simulink model "tram_sim"  (R2019b)
settings: Solver=VariableStepAuto  StartTime=0.0  StopTime=700  RelTol=1e-3
values from neighbouring files (symbols this model uses):
  B = 1/3*Te_n*1/w_b    (= 1.3022339824)    [tram.m]
  e_n = Ks*ie_max*w_b    (= 540)    [tram.m]
  g = 9.81    [tram.m]
  ie_max = 1    [tram.m]
  J = m_t*r_whl^2    (= 73.2506615098)    [tram.m]
  kb_a = 1/tau_a    (= 100)    [tram.m]
  kb_e = 1/tau_e    (= 1)    [tram.m]
  kb_spd = 1/tau_s    (= 5)    [tram.m]
  Kie = Ci_e.Ki    [tram.m]
  Kim = Cm.Ki    [tram.m]
  Kpe = Ci_e.Kp    [tram.m]
  Kpm = Cm.Kp    [tram.m]
  Ks = v_line*eta/(ie_max*w_b)    (= 1.71974522293)    [tram.m]
  La = tau_a*Ra    (= 0.00104347826087)    [tram.m]
  Le = tau_e*Re    (= 120)    [tram.m]
  m_t = m_train + m_load    (= 26000)    [tram.m]
  r_whl = s_b/w_b*10/36    (= 0.0530785562633)    [tram.m]
  Ra = (v_line-e_n)/ia_n    (= 0.104347826087)    [tram.m]
  Re = ve_max/ie_max    (= 120)    [tram.m]
  s_b = 60    [tram.m]
  Te_n = 4/3*F_tr*r_whl    (= 1226.70441142)    [tram.m]
  v_line = 600    [tram.m]
  ve_max = 120    [tram.m]
  w_b = 314    [tram.m]
undefined symbols (not defined in the file or in its folder): sigbuilder_block
settings Model: Creator=hassancurrimbhoy  LastModifiedBy=hassancurrimbhoy
settings SolverCC: ZeroCrossAlgorithm=Adaptive
settings DebuggingCC: IgnoredZcDiagnostic=none

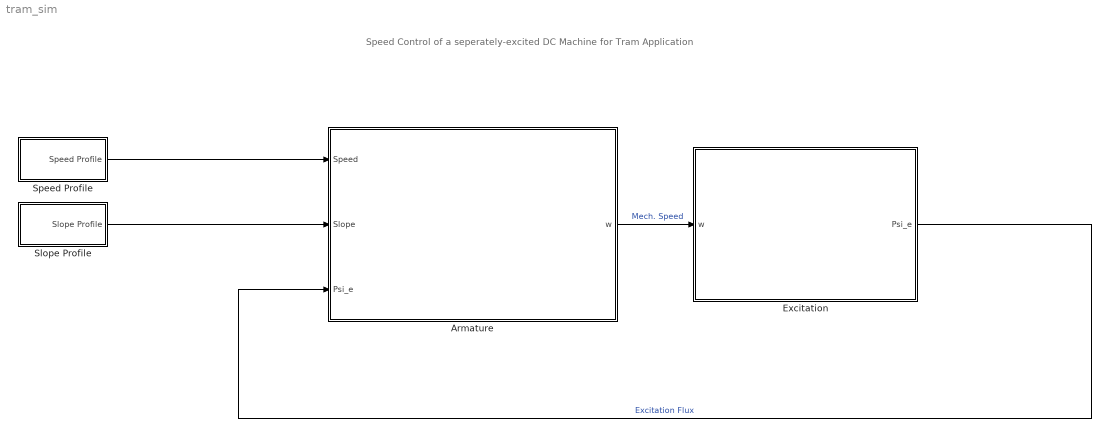
== system tram_sim ==
  note: Speed Control of a seperately-excited DC Machine for Tram Application
  Armature : Subsystem
  Excitation : Subsystem
  Slope Profile : Subsystem  Tag=STV Subsys  LoadFcn=sigbuilder_block('load');  StartFcn=sigbuilder_block('start');  StopFcn=sigbuilder_block('stop');  ClipboardFcn=sigbuilder_block('clipboard');  mask(Sigbuilder block){tuvar=[0:10]}
      mask help: Simulink:masks:SigbuilderBlock_MD
      mask init:
      | if ~strcmp(get_param(bdroot(gcbh),'SimulationStatus'),'stopped') tuvar = sigbuilder_block('maskInit'); end
      settings: CopyFcn=sigbuilder_block('copy');  DeleteFcn=sigbuilder_block('delete');  ModelCloseFcn=sigbuilder_block('modelClose');  PreSaveFcn=sigbuilder_block('preSave');  PauseFcn=sigbuilder_block('pause');  ContinueFcn=sigbuilder_block('continue');  NameChangeFcn=sigbuilder_block('namechange');  OpenFcn=sigbuilder_block('open',[437.6 199.2 550.4 400 ]);  CloseFcn=sigbuilder_block('close');
      mask Display: plot(0, 0, 100, 100,[2, 2, 32, 32, 2], [68, 8, 8, 68, 68],[32, 2], [38, 38], [32, 19, 2],[53, 60, 44], [32, 17, 17, 2],[16, 16, 31, 31]);txt = getActiveGroup(gcbh);text(2, 100, txt,'verticalAlignment', 'top');
  Speed Profile : Subsystem  Tag=STV Subsys  LoadFcn=sigbuilder_block('load');  StartFcn=sigbuilder_block('start');  StopFcn=sigbuilder_block('stop');  ClipboardFcn=sigbuilder_block('clipboard');  mask(Sigbuilder block){tuvar=[0:10]}
      mask help: Simulink:masks:SigbuilderBlock_MD
      mask init:
      | if ~strcmp(get_param(bdroot(gcbh),'SimulationStatus'),'stopped') tuvar = sigbuilder_block('maskInit'); end
      settings: CopyFcn=sigbuilder_block('copy');  DeleteFcn=sigbuilder_block('delete');  ModelCloseFcn=sigbuilder_block('modelClose');  PreSaveFcn=sigbuilder_block('preSave');  PauseFcn=sigbuilder_block('pause');  ContinueFcn=sigbuilder_block('continue');  NameChangeFcn=sigbuilder_block('namechange');  OpenFcn=sigbuilder_block('open',[437.6 199.2 550.4 400 ]);  CloseFcn=sigbuilder_block('close');
      mask Display: plot(0, 0, 100, 100,[2, 2, 32, 32, 2], [68, 8, 8, 68, 68],[32, 2], [38, 38], [32, 19, 2],[53, 60, 44], [32, 17, 17, 2],[16, 16, 31, 31]);txt = getActiveGroup(gcbh);text(2, 100, txt,'verticalAlignment', 'top');
  wires:
  Excitation/1(Psi_e) -> Armature/3(Psi_e)  "Excitation Flux"
  Armature/1(w) -> Excitation/1(w)  "Mech. Speed"
  Slope Profile/1(Slope Profile) -> Armature/2(Slope)
  Speed Profile/1(Speed Profile) -> Armature/1(Speed)

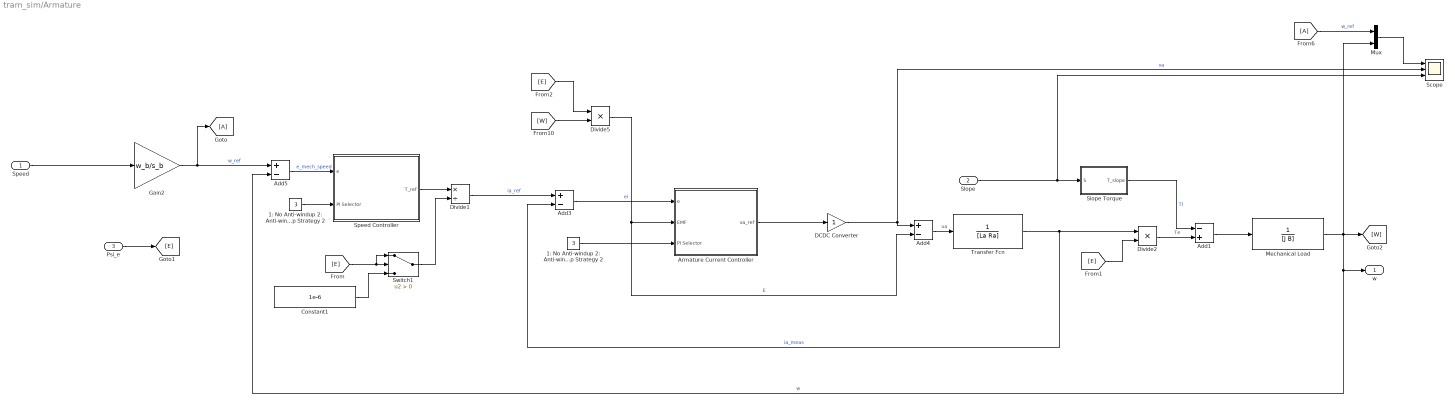
== system tram_sim/Armature ==
  Speed : Inport
  Slope : Inport  Port=2
  Psi_e : Inport  Port=3
  1: No Anti-windup 2: Anti-windup Stragtegy 1 3: Anti-windup Strategy 2 : Constant  Value=3
  1: No Anti-windup 2: Anti-windup Strategy 1 3: Anti-windup Strategy 2 : Constant  Value=3
  Add1 : Sum  Inputs=-+
  Add3 : Sum  Inputs=+-
  Add4 : Sum  Inputs=+-
  Add5 : Sum  Inputs=+-
  Armature Current Controller : Subsystem
  Constant1 : Constant  Value=1e-6
  DCDC Converter : Gain
  Divide1 : Product  Inputs=*/
  Divide2 : Product  Inputs=**
  Divide5 : Product  Inputs=**
  Gain2 : Gain  Gain=w_b/s_b
  Mechanical Load : TransferFcn  Denominator=[J B]
  Mux : Mux  Inputs=2
  Scope : Scope  NumInputPorts=3
  Slope Torque : Subsystem
  Speed Controller : Subsystem
  Switch1 : Switch  Criteria=u2 > Threshold
  Transfer Fcn : TransferFcn  Denominator=[La Ra]
  w : Outport
  wires:
  1: No Anti-windup 2: Anti-windup Stragtegy 1 3: Anti-windup Strategy 2/1 -> Speed Controller/2(PI Selector)
  Armature Current Controller/1("va_ref ") -> DCDC Converter/1
  Constant1/1 -> Switch1/3
  Add1/1 -> Mechanical Load/1
  Gain2/1 -> Add5/1, [A]  "w_ref"
  Mechanical Load/1 -> Mux/2, [W], w/1, Add5/2  "w"
  [A] -> Mux/1  "w_ref"
  [W] -> Divide5/2
  Mux/1 -> Scope/1
  Slope Torque/1(T_slope) -> Add1/1  "Tl"
  Add5/1 -> Speed Controller/1(e)  "e_mech_speed"
  Speed Controller/1("T_ref ") -> Divide1/1
  DCDC Converter/1 -> Scope/2, Add4/1  "va"
  Divide2/1 -> Add1/2  "Te"
  Add3/1 -> Armature Current Controller/1(e)  "ei"
  Add4/1 -> Transfer Fcn/1  "ua"
  [E] -> Divide2/2
  1: No Anti-windup 2: Anti-windup Strategy 1 3: Anti-windup Strategy 2/1 -> Armature Current Controller/3("PI Selector ")
  Divide1/1 -> Add3/1  "ia_ref"
  Divide5/1 -> Add4/2, Armature Current Controller/2(EMF)  "E"
  [E] -> Switch1/1, Switch1/2
  Transfer Fcn/1 -> Divide2/1, Add3/2  "ia_meas"
  Psi_e/1 -> [E]
  [E] -> Divide5/1
  Speed/1 -> Gain2/1
  Slope/1 -> Scope/3, Slope Torque/1(S)
  Switch1/1 -> Divide1/2

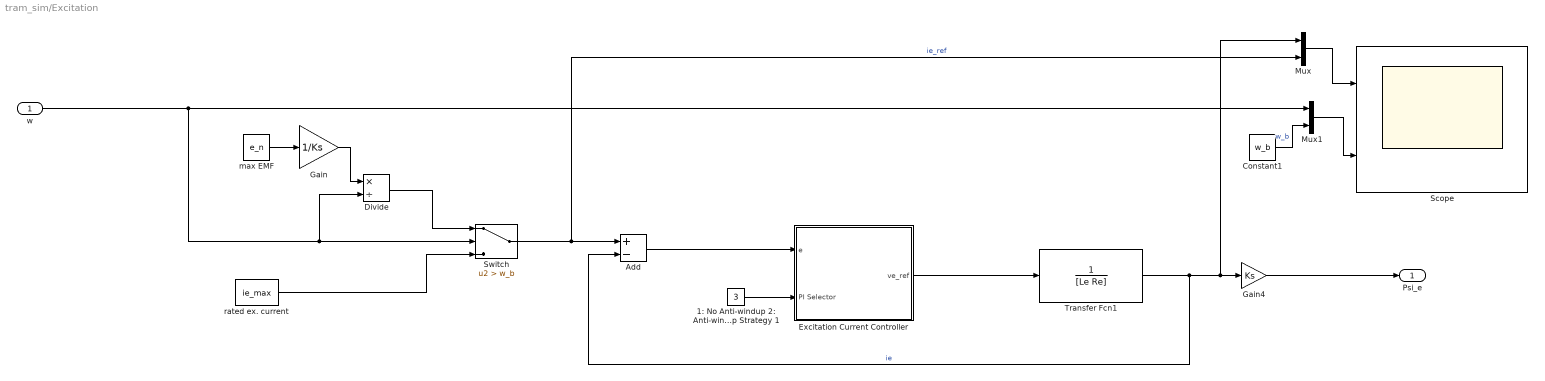
== system tram_sim/Excitation ==
  w : Inport
  1: No Anti-windup 2: Anti-windup Strategy 1 3: Anti-windup Strategy 1 : Constant  Value=3
  Add : Sum  Inputs=+-
  Constant1 : Constant  Value=w_b
  Divide : Product  Inputs=*/
  Excitation Current Controller : Subsystem
  Gain : Gain  Gain=1/Ks
  Gain4 : Gain  Gain=Ks
  Mux : Mux  Inputs=2
  Mux1 : Mux  Inputs=2
  Scope : Scope  NumInputPorts=2
  Switch : Switch  Criteria=u2 > Threshold  Threshold=w_b
  Transfer Fcn1 : TransferFcn  Denominator=[Le Re]
  max EMF : Constant  Value=e_n
  rated ex. current : Constant  Value=ie_max
  Psi_e : Outport
  wires:
  Excitation Current Controller/1("ve_ref ") -> Transfer Fcn1/1
  Add/1 -> Excitation Current Controller/1(e)
  Gain/1 -> Divide/1
  Transfer Fcn1/1 -> Mux/1, Gain4/1, Add/2  "ie"
  rated ex. current/1 -> Switch/3
  1: No Anti-windup 2: Anti-windup Strategy 1 3: Anti-windup Strategy 1/1 -> Excitation Current Controller/2("PI Selector ")
  Switch/1 -> Mux/2, Add/1  "ie_ref"
  Divide/1 -> Switch/1
  max EMF/1 -> Gain/1
  w/1 -> Switch/2, Divide/2, Mux1/1
  Mux/1 -> Scope/1
  Constant1/1 -> Mux1/2  "w_b"
  Mux1/1 -> Scope/2
  Gain4/1 -> Psi_e/1

== system tram_sim/Slope Profile ==
  Demux : Demux  Tag=STV Demux  Outputs=1
  FromWs : FromWorkspace  Tag=STV FromWs  VariableName=tuvar  SampleTime=0
      SigBuilderData=|
      | common.afterFinalStr = 'Extrapolate'
      | common.sampleTime = 0
      | dataSet.timeRange = [0 700]
      | dataSet.name = 'Group 1'
      | sbobj.Groups.Name = 'Group 1'
      | sbobj.Groups.Signals.Name = 'Slope Profile'
      | sbobj.Groups.Signals.XData = [0 1 2 3 4 5 6 7 8 9 10 11 ... (662 elements, 1x662)]
      | sbobj.Groups.Signals.YData = [0 0 0 0 0 0 0 0 0 0 0 0 0 0 0 0 0 0 0 0 0 0 0 0 0 0 0 0 0 0 0 0 0 0 0 0 0 0 0 0 0 0 0 0 0 0 0 0 0 0 0 0 0 0 0 0 0 0 0 0 0 0 0 0 0 0 0 0 0 0 0 0 0 0 0 0 0 0 0 0 0 0 0 0 0 0 0 0 0 0 0 0 0 0 0 0 0 0 0 0 0 0 0 0 0 0 0 0 0 0 0 0 0 0 0 0 0 0 0 0 0 0 0 0 0 0 0 0 0 0 0 0 0 0 0 0 0 0 0 0 0 0 0 0 0 0 0 0 0 0 0 0 0 0 0 0 0 0 0 0 0 0 0 0 0 0 0 0 0 0 0 0 0 0 0 0 0 0 0 0 0 0 0 0 0 0 0 0 0 0 0 0 0 0 0 0 0 0 0 0 0 0 0 0 0 0 0 0 0 0 0 0 0 0 0 0 0 0 0 0 0 0 0 5 5 5 5 5 5 5 5 5 5 5 5 5 5 5 5 5 5 5 5 5 5 5 5 5 5 5 5 5 5 5 5 5 5 5 5 5 5 5 5 5 5 5 5 5 5 5 5 5 5 5 5 5 5 5 5 5 5 5 5 0 0 0 0 0 0 0 0 0 0 0 0 0 0 0 0 0 0 0 0 0 0 0 0 0 0 0 0 0 0 0 0 0 0 0 0 0 0 0 0 0 0 0 0 0 0 0 0 0 0 0 0 0 0 0 0 0 0 0 0 0 0 0 0 0 0 0 0 0 0 0 0 0 0 0 0 0 0 0 0 0 0 0 0 0 0 0 0 0 0 0 0 0 0 0 0 0 0 0 0 0 0 0 0 0 0 0 0 0 0 0 0 0 0 0 0 0 0 0 0 0 0 0 0 0 0 0 0 0 0 0 0 0 0 0 0 0 0 0 0 0 0 0 0 0 0 0 0 0 0 0 0 0 0 0 0 0 0 0 0 0 0 0 0 0 0 0 0 0 0 0 0 0 0 0 0 0 0 0 0 0 0 0 0 0 0 0 0 0 0 0 0 0 0 0 0 0 0 0 0 0 0 0 0 0 0 0 0 0 0 0 0 0 0 0 0 -5 -5 -5 -5 -5 -5 -5 -5 -5 -5 -5 -5 -5 -5 -5 -5 -5 -5 -5 -5 -5 -5 -5 -5 -5 -5 -5 -5 -5 -5 -5 -5 -5 -5 -5 -5 -5 -5 -5 -5 -5 -5 -5 -5 -5 -5 -5 -5 -5 -5 -5 -5 -5 -5 -5 -5 -5 -5 -5 -5 0 0 0 0 0 0 0 0 0 0 0 0 0 0 0 0 0 0 0 0 0 0 0 0 0 0 0 0 0 0 0 0 0 0 0 0 0 0 0 0 0 0 0 0 0 0 0 0 0 0 0 0 0 0 0 0 0 0 0 0 0 0 0 0 0 0 0 0 0 0 0 0 0 0 0 0 0 0 0 0 0 0 0 0 0 0 0 0 0 0 0 0 0 0 0 0 0 0 0 0 0 0 0]
      | sbobj.Groups.TimeRange = [0 700]
  Slope Profile : Outport  Tag=STV Outport
  wires:
  FromWs/1 -> Demux/1
  Demux/1 -> Slope Profile/1

== system tram_sim/Speed Profile ==
  Demux : Demux  Tag=STV Demux  Outputs=1
  FromWs : FromWorkspace  Tag=STV FromWs  VariableName=tuvar  SampleTime=0
      SigBuilderData=|
      | common.afterFinalStr = 'Extrapolate'
      | common.sampleTime = 0
      | dataSet.timeRange = [0 700]
      | dataSet.name = 'Group 1'
      | sbobj.Groups.Name = 'Group 1'
      | sbobj.Groups.Signals.Name = 'Speed Profile'
      | sbobj.Groups.Signals.XData = [0 1 2 3 4 5 6 7 8 9 10 11 ... (662 elements, 1x662)]
      | sbobj.Groups.Signals.YData = [35 35 35 35 35 35 35 35 35 35 35 35 35 35 35 35 35 35 35 35 35 35 35 35 35 35 35 35 35 35 35 35 35 35 35 35 35 35 35 35 35 35 35 35 35 35 35 35 35 35 35 35 35 35 35 35 35 35 35 35 35 35 35 35 35 35 35 35 35 35 35 35 35 35 35 35 35 35 35 35 35 35 35 35 35 35 35 35 35 35 35 35 35 35 35 35 35 35 35 35 35 35 35 60 60 60 60 60 60 60 60 60 60 60 60 60 60 60 60 60 60 60 60 60 60 60 60 60 60 60 60 60 60 60 60 60 60 60 60 60 60 60 60 60 60 60 60 60 60 60 60 60 60 60 60 60 60 60 60 60 60 60 60 60 60 60 60 60 60 60 60 60 60 60 60 60 60 60 60 60 60 60 60 60 60 60 60 60 60 60 60 60 60 60 60 60 60 60 60 60 60 60 60 60 60 60 60 60 60 60 60 60 60 60 60 60 60 60 60 60 60 60 60 60 60 60 60 60 60 60 60 60 60 60 60 60 60 60 60 60 60 60 60 60 60 60 60 60 60 60 60 60 60 60 60 60 60 60 60 60 60 60 60 60 60 60 60 60 60 60 60 60 60 60 60 60 60 60 60 60 60 60 60 75 75 75 75 75 75 75 75 75 75 75 75 75 75 75 75 75 75 75 75 75 75 75 75 75 75 75 75 75 75 75 75 75 75 75 75 75 75 75 75 75 75 75 75 75 75 75 75 75 75 75 75 75 75 75 75 75 75 75 75 75 75 75 75 75 75 75 75 75 75 75 75 75 75 75 75 75 75 75 75 75 75 75 75 75 75 75 75 75 75 75 75 75 75 75 75 60 60 60 60 60 60 60 60 60 60 60 60 60 60 60 60 60 60 60 60 60 60 60 60 60 60 60 60 60 60 60 60 60 60 60 60 60 60 60 60 60 60 60 60 60 60 60 60 60 60 60 60 60 60 60 60 60 60 60 60 60 60 60 60 60 60 60 60 60 60 60 60 60 60 60 60 60 60 60 60 60 60 60 60 60 60 60 60 60 60 60 60 60 60 60 60 60 60 60 60 60 60 60 60 60 60 60 60 60 60 60 60 60 60 60 60 60 60 60 60 60 60 60 60 60 60 60 60 60 60 60 60 60 60 60 60 60 60 60 60 60 60 60 60 60 60 60 60 60 60 60 60 60 60 60 60 60 60 60 60 60 60 60 60 60 60 60 60 60 60 60 60 60 60 60 60 60 60 60 60 35 35 35 35 35 35 35 35 35 35 35 35 35 35 35 35 35 35 35 35 35 35 35 35 35 35 35 35 35 35 35 35 35 35 35 35 35 35 35 35 35 35 35 35 35 35 35 35 35 35 35 35 35 35 35 35 35 35 35 35 35 35 35 35 35 35 35 35 35 35 35 35 35 35 35 35 35 35 35 35 35 35 35 35 35 35 35 35 35 35 35 35 35 35 35 35 35 35 35 35 35 35 35]
      | sbobj.Groups.TimeRange = [0 700]
  Speed Profile : Outport  Tag=STV Outport
  wires:
  FromWs/1 -> Demux/1
  Demux/1 -> Speed Profile/1

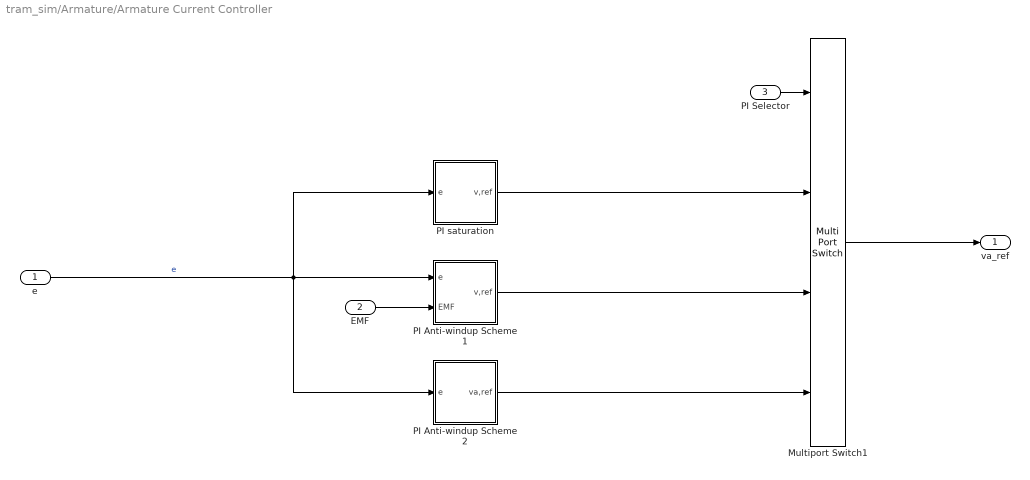
== system tram_sim/Armature/Armature Current Controller ==
  e : Inport
  EMF : Inport  Port=2
  "PI Selector " : Inport  Port=3
  Multiport Switch1 : MultiPortSwitch
  PI Anti-windup Scheme 1 : Subsystem
  PI Anti-windup Scheme 2 : Subsystem
  PI saturation : Subsystem
  "va_ref " : Outport
  wires:
  PI saturation/1(v,ref) -> Multiport Switch1/2
  PI Anti-windup Scheme 2/1(va,ref) -> Multiport Switch1/4
  e/1 -> PI Anti-windup Scheme 1/1(e), PI Anti-windup Scheme 2/1(e), PI saturation/1(e)  "e"
  PI Anti-windup Scheme 1/1(v,ref) -> Multiport Switch1/3
  "PI Selector "/1 -> Multiport Switch1/1
  Multiport Switch1/1 -> "va_ref "/1
  EMF/1 -> PI Anti-windup Scheme 1/2(EMF)

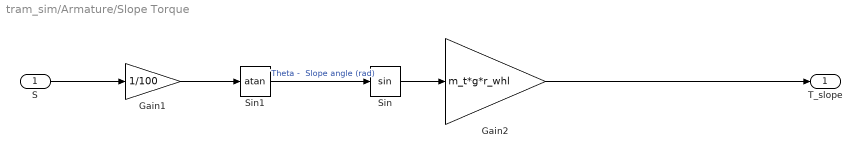
== system tram_sim/Armature/Slope Torque ==
  S : Inport
  Gain1 : Gain  Gain=1/100
  Gain2 : Gain  Gain=m_t*g*r_whl
  Sin : Trigonometry
  Sin1 : Trigonometry  Operator=atan
  T_slope : Outport
  wires:
  Sin/1 -> Gain2/1
  S/1 -> Gain1/1
  Sin1/1 -> Sin/1  "Theta -  Slope angle (rad)"
  Gain1/1 -> Sin1/1
  Gain2/1 -> T_slope/1

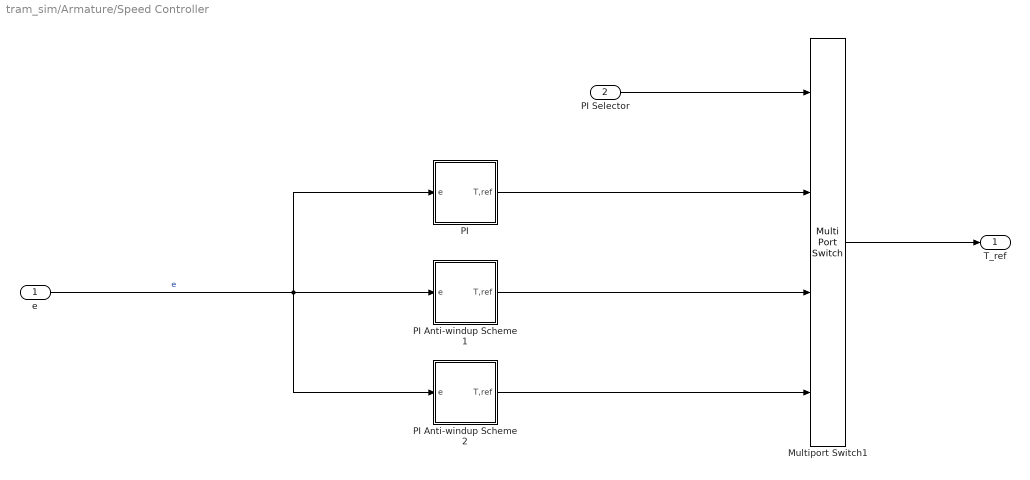
== system tram_sim/Armature/Speed Controller ==
  e : Inport
  PI Selector : Inport  Port=2
  Multiport Switch1 : MultiPortSwitch
  PI : Subsystem
  PI Anti-windup Scheme 1 : Subsystem
  PI Anti-windup Scheme 2 : Subsystem
  "T_ref " : Outport
  wires:
  PI Anti-windup Scheme 1/1(T,ref) -> Multiport Switch1/3
  e/1 -> PI/1(e), PI Anti-windup Scheme 1/1(e), PI Anti-windup Scheme 2/1(e)  "e"
  Multiport Switch1/1 -> "T_ref "/1
  PI/1(T,ref) -> Multiport Switch1/2
  PI Selector/1 -> Multiport Switch1/1
  PI Anti-windup Scheme 2/1(T,ref) -> Multiport Switch1/4

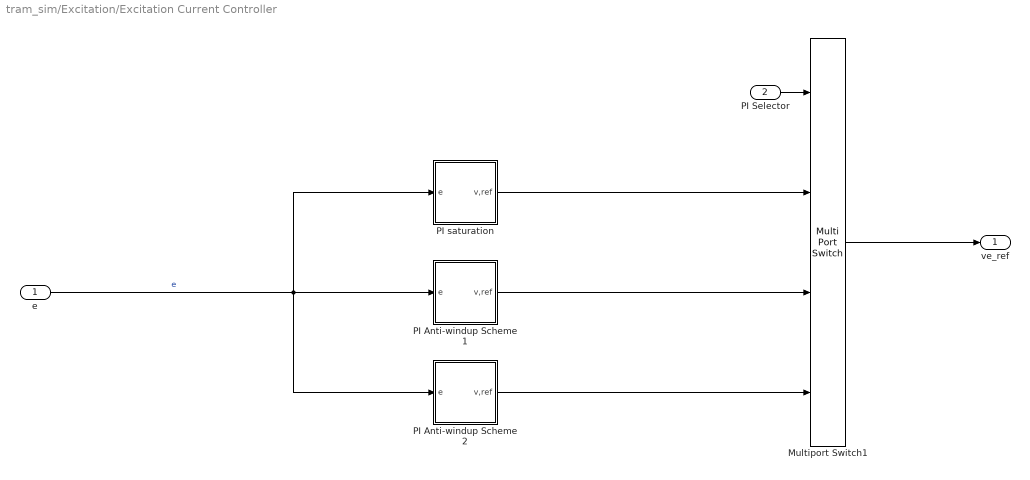
== system tram_sim/Excitation/Excitation Current Controller ==
  e : Inport
  "PI Selector " : Inport  Port=2
  Multiport Switch1 : MultiPortSwitch
  PI Anti-windup Scheme 1 : Subsystem
  PI Anti-windup Scheme 2 : Subsystem
  PI saturation : Subsystem
  "ve_ref " : Outport
  wires:
  PI saturation/1(v,ref) -> Multiport Switch1/2
  PI Anti-windup Scheme 2/1(v,ref) -> Multiport Switch1/4
  e/1 -> PI saturation/1(e), PI Anti-windup Scheme 1/1(e), PI Anti-windup Scheme 2/1(e)  "e"
  PI Anti-windup Scheme 1/1(v,ref) -> Multiport Switch1/3
  "PI Selector "/1 -> Multiport Switch1/1
  Multiport Switch1/1 -> "ve_ref "/1

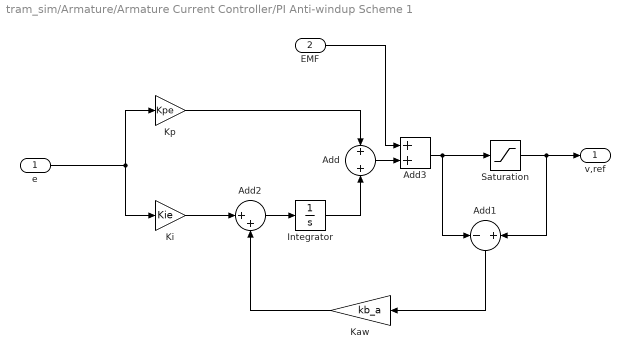
== system tram_sim/Armature/Armature Current Controller/PI Anti-windup Scheme 1 ==
  e : Inport
  EMF : Inport  Port=2
  Add : Sum
  Add1 : Sum  Inputs=-+
  Add2 : Sum  Inputs=|++
  Add3 : Sum
  Integrator : Integrator
  Kaw : Gain  Gain=kb_a
  Ki : Gain  Gain=Kie
  Kp : Gain  Gain=Kpe
  Saturation : Saturate  UpperLimit=v_line  LowerLimit=-v_line
  v,ref : Outport
  wires:
  Ki/1 -> Add2/1
  Kp/1 -> Add/1
  Integrator/1 -> Add/2
  e/1 -> Ki/1, Kp/1
  Saturation/1 -> Add1/2, v,ref/1
  Add2/1 -> Integrator/1
  Add1/1 -> Kaw/1
  Kaw/1 -> Add2/2
  Add/1 -> Add3/2
  Add3/1 -> Add1/1, Saturation/1
  EMF/1 -> Add3/1

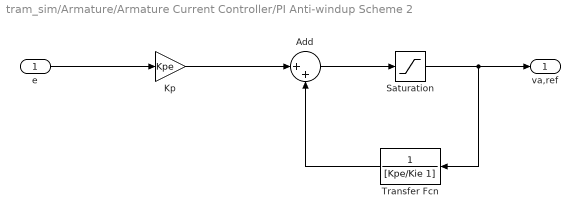
== system tram_sim/Armature/Armature Current Controller/PI Anti-windup Scheme 2 ==
  e : Inport
  Add : Sum  Inputs=|++
  Kp : Gain  Gain=Kpe
  Saturation : Saturate  UpperLimit=v_line  LowerLimit=-v_line
  Transfer Fcn : TransferFcn  Denominator=[Kpe/Kie 1]
  va,ref : Outport
  wires:
  Kp/1 -> Add/1
  e/1 -> Kp/1
  Transfer Fcn/1 -> Add/2
  Add/1 -> Saturation/1
  Saturation/1 -> Transfer Fcn/1, va,ref/1

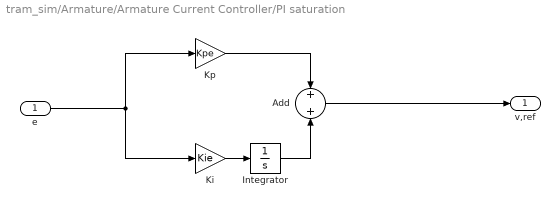
== system tram_sim/Armature/Armature Current Controller/PI saturation ==
  e : Inport
  Add : Sum
  Integrator : Integrator
  Ki : Gain  Gain=Kie
  Kp : Gain  Gain=Kpe
  v,ref : Outport
  wires:
  Ki/1 -> Integrator/1
  Kp/1 -> Add/1
  Integrator/1 -> Add/2
  e/1 -> Ki/1, Kp/1
  Add/1 -> v,ref/1

== system tram_sim/Armature/Speed Controller/PI ==
  e : Inport
  Add : Sum
  Integrator : Integrator
  Ki : Gain  Gain=Kim
  Kp : Gain  Gain=Kpm
  T,ref : Outport
  wires:
  Ki/1 -> Integrator/1
  Kp/1 -> Add/1
  Integrator/1 -> Add/2
  e/1 -> Ki/1, Kp/1
  Add/1 -> T,ref/1

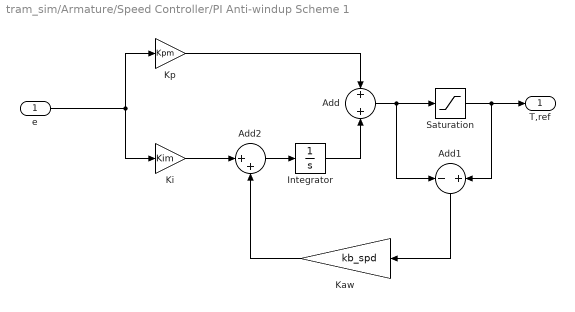
== system tram_sim/Armature/Speed Controller/PI Anti-windup Scheme 1 ==
  e : Inport
  Add : Sum
  Add1 : Sum  Inputs=-+
  Add2 : Sum  Inputs=|++
  Integrator : Integrator
  Kaw : Gain  Gain=kb_spd
  Ki : Gain  Gain=Kim
  Kp : Gain  Gain=Kpm
  Saturation : Saturate  UpperLimit=Te_n  LowerLimit=-Te_n
  T,ref : Outport
  wires:
  Ki/1 -> Add2/1
  Kp/1 -> Add/1
  Add/1 -> Add1/1, Saturation/1
  Integrator/1 -> Add/2
  e/1 -> Ki/1, Kp/1
  Saturation/1 -> Add1/2, T,ref/1
  Add2/1 -> Integrator/1
  Add1/1 -> Kaw/1
  Kaw/1 -> Add2/2

== system tram_sim/Armature/Speed Controller/PI Anti-windup Scheme 2 ==
  e : Inport
  Add : Sum  Inputs=|++
  Kp : Gain  Gain=Kpm
  Saturation : Saturate  UpperLimit=Te_n  LowerLimit=-Te_n
  Transfer Fcn : TransferFcn  Denominator=[Kpm/Kim 1]
  T,ref : Outport
  wires:
  Kp/1 -> Add/1
  e/1 -> Kp/1
  Add/1 -> Saturation/1
  Transfer Fcn/1 -> Add/2
  Saturation/1 -> Transfer Fcn/1, T,ref/1

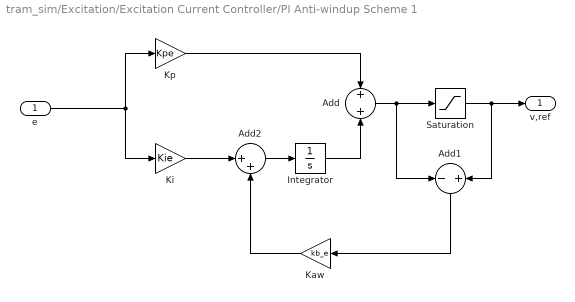
== system tram_sim/Excitation/Excitation Current Controller/PI Anti-windup Scheme 1 ==
  e : Inport
  Add : Sum
  Add1 : Sum  Inputs=-+
  Add2 : Sum  Inputs=|++
  Integrator : Integrator
  Kaw : Gain  Gain=kb_e
  Ki : Gain  Gain=Kie
  Kp : Gain  Gain=Kpe
  Saturation : Saturate  UpperLimit=ve_max  LowerLimit=-ve_max
  v,ref : Outport
  wires:
  Ki/1 -> Add2/1
  Kp/1 -> Add/1
  Add/1 -> Add1/1, Saturation/1
  Integrator/1 -> Add/2
  e/1 -> Ki/1, Kp/1
  Saturation/1 -> Add1/2, v,ref/1
  Add2/1 -> Integrator/1
  Add1/1 -> Kaw/1
  Kaw/1 -> Add2/2

== system tram_sim/Excitation/Excitation Current Controller/PI Anti-windup Scheme 2 ==
  e : Inport
  Add : Sum  Inputs=|++
  Kp : Gain  Gain=Kpe
  Saturation : Saturate  UpperLimit=ve_max  LowerLimit=-ve_max
  Transfer Fcn : TransferFcn  Denominator=[Kpe/Kie 1]
  v,ref : Outport
  wires:
  Kp/1 -> Add/1
  e/1 -> Kp/1
  Add/1 -> Saturation/1
  Transfer Fcn/1 -> Add/2
  Saturation/1 -> Transfer Fcn/1, v,ref/1

== system tram_sim/Excitation/Excitation Current Controller/PI saturation ==
  e : Inport
  Add : Sum
  Integrator : Integrator
  Ki : Gain  Gain=Kie
  Kp : Gain  Gain=Kpe
  v,ref : Outport
  wires:
  Ki/1 -> Integrator/1
  Kp/1 -> Add/1
  Integrator/1 -> Add/2
  e/1 -> Ki/1, Kp/1
  Add/1 -> v,ref/1
